simulink model "N_scheme_RP4"  (R2024b)
settings: Solver=VariableStepAuto  StartTime=0.0  StopTime=10.0  RelTol=1e-3
values from neighbouring files (symbols this model uses):
  b_n = (b_max + b_min)/2    (= 84)    [P15.m]
  c = 0.707    [P15.m]
  Ga = -100    [P15.m]
  Gf = 1/(Kd*Gs)    (= 0.333333333333)    [P15.m]
  Gs = 3    [P15.m]
  K_n = (K_max + K_min)/2    (= 40)    [P15.m]
  Wb = (b_max - b_min)/2    (= 36)    [P15.m]
  Wk = (K_max - K_min)/2    (= 20)    [P15.m]
libraries: cstblocks x2
settings Model: Creator=adrian  LastModifiedBy=adrian

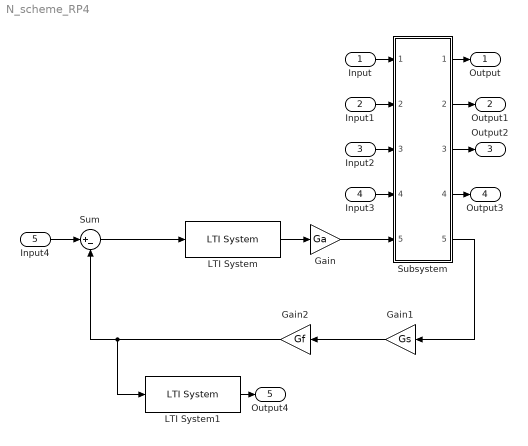
== system N_scheme_RP4 ==
  Input : Inport
  Input1 : Inport  Port=2
  Input2 : Inport  Port=3
  Input3 : Inport  Port=4
  Input4 : Inport  Port=5
  Gain : Gain  Gain=Ga
  Gain1 : Gain  Gain=Gs
  Gain2 : Gain  Gain=Gf
  LTI System : cstblocks/LTI System  sys=Gc  IC=[]  PadeOrder=0
  LTI System1 : cstblocks/LTI System  sys=WT_mu_RP4  IC=[]  PadeOrder=0
  Subsystem : Subsystem
  Sum : Sum  Inputs=|+-
  Output : Outport
  Output1 : Outport  Port=2
  Output2 : Outport  Port=3
  Output3 : Outport  Port=4
  Output4 : Outport  Port=5
  wires:
  Gain/1 -> Subsystem/5(Input4)
  LTI System/1 -> Gain/1
  Gain1/1 -> Gain2/1
  Subsystem/5(Output4) -> Gain1/1
  Sum/1 -> LTI System/1
  Gain2/1 -> LTI System1/1, Sum/2
  Input2/1 -> Subsystem/3(Input2)
  Input1/1 -> Subsystem/2(Input1)
  Input/1 -> Subsystem/1(Input)
  Input3/1 -> Subsystem/4(Input3)
  Subsystem/1(Output) -> Output/1
  Subsystem/2(Output1) -> Output1/1
  Subsystem/3(Output2) -> Output2/1
  Subsystem/4(Output3) -> Output3/1
  Input4/1 -> Sum/1
  LTI System1/1 -> Output4/1

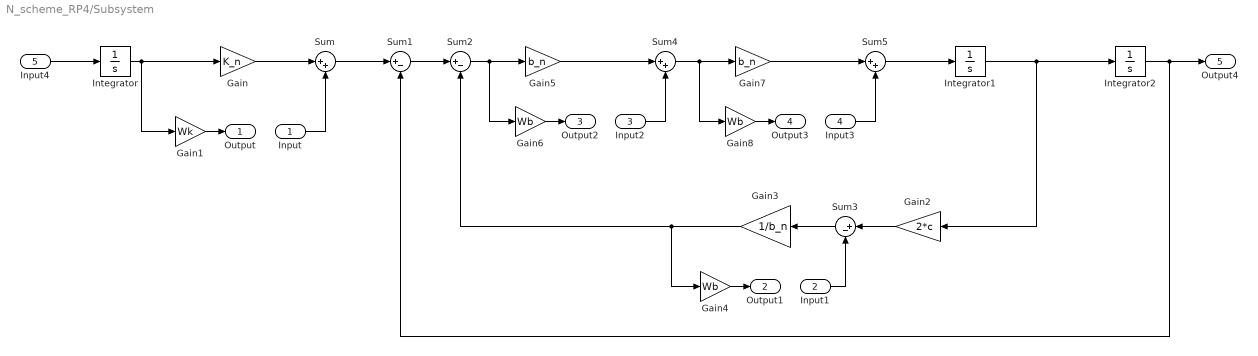
== system N_scheme_RP4/Subsystem ==
  Input : Inport
  Input1 : Inport  Port=2
  Input2 : Inport  Port=3
  Input3 : Inport  Port=4
  Input4 : Inport  Port=5
  Gain : Gain  Gain=K_n
  Gain1 : Gain  Gain=Wk
  Gain2 : Gain  Gain=2*c
  Gain3 : Gain  Gain=1/b_n
  Gain4 : Gain  Gain=Wb
  Gain5 : Gain  Gain=b_n
  Gain6 : Gain  Gain=Wb
  Gain7 : Gain  Gain=b_n
  Gain8 : Gain  Gain=Wb
  Integrator : Integrator
  Integrator1 : Integrator
  Integrator2 : Integrator
  Sum : Sum  Inputs=|++
  Sum1 : Sum  Inputs=|+-
  Sum2 : Sum  Inputs=|+-
  Sum3 : Sum  Inputs=|+-
  Sum4 : Sum  Inputs=|++
  Sum5 : Sum  Inputs=|++
  Output : Outport
  Output1 : Outport  Port=2
  Output2 : Outport  Port=3
  Output3 : Outport  Port=4
  Output4 : Outport  Port=5
  wires:
  Integrator/1 -> Gain1/1, Gain/1
  Gain/1 -> Sum/1
  Gain1/1 -> Output/1
  Input/1 -> Sum/2
  Sum/1 -> Sum1/1
  Sum1/1 -> Sum2/1
  Integrator1/1 -> Gain2/1, Integrator2/1
  Gain2/1 -> Sum3/1
  Sum3/1 -> Gain3/1
  Gain3/1 -> Sum2/2, Gain4/1
  Gain4/1 -> Output1/1
  Input1/1 -> Sum3/2
  Sum2/1 -> Gain6/1, Gain5/1
  Gain6/1 -> Output2/1
  Input2/1 -> Sum4/2
  Gain5/1 -> Sum4/1
  Gain7/1 -> Sum5/1
  Input3/1 -> Sum5/2
  Gain8/1 -> Output3/1
  Sum4/1 -> Gain7/1, Gain8/1
  Sum5/1 -> Integrator1/1
  Integrator2/1 -> Output4/1, Sum1/2
  Input4/1 -> Integrator/1
